simulink model "PID_control_simulink"  (R2020a)
settings: Solver=FixedStepAuto  StartTime=0.0  StopTime=600  FixedStep=1  RelTol=1e-3
values from neighbouring files (symbols this model uses):
  K = 0.7087    [PD_control_1.m]    (also in PD_control_2.m; PID_control_1.m = 0.7243; PID_control_2.m = 0.7243; PI_control_1.m)
  Kp = (1/K)*(T/L)*(1.25 + L/(6*T))    (= 7.94369684431)    [PD_control_1.m]    (also in PD_control_2.m; PID_control_1.m = 8.38060708808; PID_control_2.m = 8.38060708808; PI_control_1.m = 5.667723804)
  L = 33.8800    (= 33.88)    [PD_control_1.m]    (also in PD_control_2.m; PID_control_1.m = 33.398; PID_control_2.m = 33.398; PI_control_1.m)
  T = 148.0700    (= 148.07)    [PD_control_1.m]    (also in PD_control_2.m; PID_control_1.m = 162.4602; PID_control_2.m = 162.4602; PI_control_1.m)
  Td = L*((6*T - 2*L)/(22*T + 3*L))    (= 8.27700831751)    [PD_control_1.m]    (also in PD_control_2.m; PID_control_1.m = 12.8256849784; PID_control_2.m = 12.8256849784)
  Ti = 1/((0.842/T)*((L/T)^(-0.738)))    (= 60.0356639465)    [PID_control_1.m]    (also in PID_control_2.m; PI_control_1.m = 76.5792527223; PI_control_2.m = 76.5792527223)
  y_initial = TCLab_data.T1(1)    [PD_control_2.m]    (also in PID_control_2.m; PI_control_2.m; P_control_2.m)
settings Model: Creator=itsri  LastModifiedBy=pedro_000
settings DataIOCC: ReturnWorkspaceOutputs=off

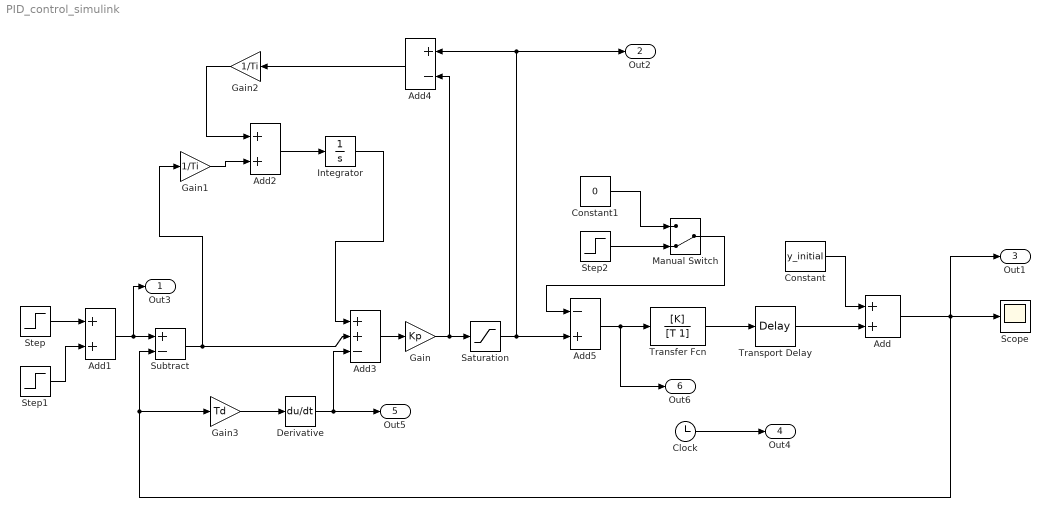
== system PID_control_simulink ==
  Add : Sum
  Add1 : Sum
  Add2 : Sum
  Add3 : Sum  Inputs=++-
  Add4 : Sum  Inputs=+-
  Add5 : Sum  Inputs=-+
  Clock : Clock
  Constant : Constant  Value=y_initial
  Constant1 : Constant  Value=0
  Derivative : Derivative
  Gain : Gain  Gain=Kp
  Gain1 : Gain  Gain=1/Ti
  Gain2 : Gain  Gain=1/Ti
  Gain3 : Gain  Gain=Td
  Integrator : Integrator
  Manual Switch : ManualSwitch  CurrentSetting=0
  Saturation : Saturate  UpperLimit=100  LowerLimit=0
  Scope : Scope
  Step : Step  Time=0  After=30  SampleTime=0
  Step1 : Step  Time=200  After=30  SampleTime=0
  Step2 : Step  Time=400  After=40  SampleTime=0
  Subtract : Sum  Inputs=+-
  Transfer Fcn : TransferFcn  Numerator=[K]  Denominator=[T 1]
  Transport Delay : TransportDelay  DelayTime=L
  Out3 : Outport
  Out2 : Outport  Port=2
  Out1 : Outport  Port=3
  Out4 : Outport  Port=4
  Out5 : Outport  Port=5
  Out6 : Outport  Port=6
  wires:
  Clock/1 -> Out4/1
  Gain/1 -> Add4/2, Saturation/1
  Saturation/1 -> Add5/2, Out2/1, Add4/1
  Transport Delay/1 -> Add/2
  Constant/1 -> Add/1
  Add/1 -> Gain3/1, Subtract/2, Scope/1, Out1/1
  Subtract/1 -> Add3/2, Gain1/1
  Add1/1 -> Out3/1, Subtract/1
  Step/1 -> Add1/1
  Step1/1 -> Add1/2
  Gain1/1 -> Add2/2
  Add3/1 -> Gain/1
  Add2/1 -> Integrator/1
  Integrator/1 -> Add3/1
  Add4/1 -> Gain2/1
  Gain2/1 -> Add2/1
  Add5/1 -> Out6/1, Transfer Fcn/1
  Constant1/1 -> Manual Switch/1
  Step2/1 -> Manual Switch/2
  Manual Switch/1 -> Add5/1
  Transfer Fcn/1 -> Transport Delay/1
  Derivative/1 -> Out5/1, Add3/3
  Gain3/1 -> Derivative/1
